simulink model "Lab4_LeadTF"  (R2016a)
settings: Solver=VariableStepAuto  StartTime=0.0  StopTime=10.0  FixedStep=.00  MaxStep=.001  RelTol=1e-3
settings Model: Creator=jordan  LastModifiedBy=jordan

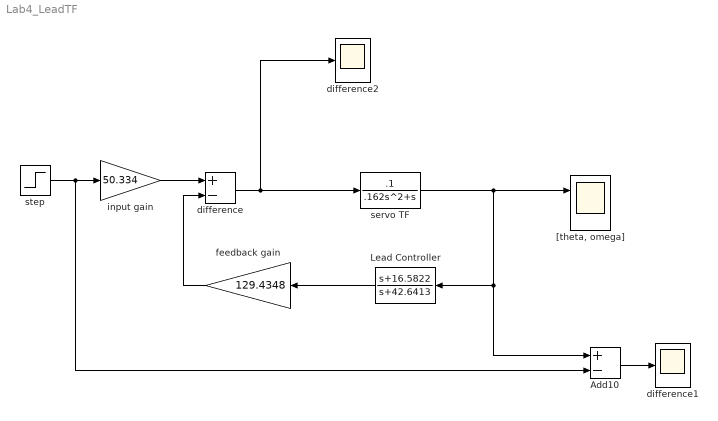
== system Lab4_LeadTF ==
  Add10 : Sum  Inputs=+-
  Lead Controller : TransferFcn  Numerator=[1 16.5822]  Denominator=[1 42.6413]
  "[theta, omega]" : Scope  NumInputPorts=2
  difference : Sum  Inputs=+-
  difference1 : Scope
  difference2 : Scope
  feedback gain : Gain  Gain=129.4348
  input gain : Gain  Gain=50.334
  servo TF : TransferFcn  Numerator=[.1]  Denominator=[.162 1 0]
  step : Step  SampleTime=0
  wires:
  step/1 -> Add10/2, input gain/1
  feedback gain/1 -> difference/2
  Lead Controller/1 -> feedback gain/1
  input gain/1 -> difference/1
  Add10/1 -> difference1/1
  difference/1 -> servo TF/1, difference2/1
  servo TF/1 -> Add10/1, Lead Controller/1, "[theta, omega]"/1
